simulink model "P1_RC_SIMULINK"  (R2022b)
settings: Solver=VariableStepAuto  StartTime=0.0  StopTime=2.350  RelTol=1e-3
values from neighbouring files (symbols this model uses):
  alpha = (-1)/tau    (= -2.12765957447)    [Main.m]    (also in P1_DINAMICA_SISTEMAS.m)
  beta = 1/tau    (= 2.12765957447)    [Main.m]    (also in P1_DINAMICA_SISTEMAS.m)
  y0 = 2    [Main.m]    (also in P1_DINAMICA_SISTEMAS.m)
settings Model: Creator=zamor  LastModifiedBy=zamor

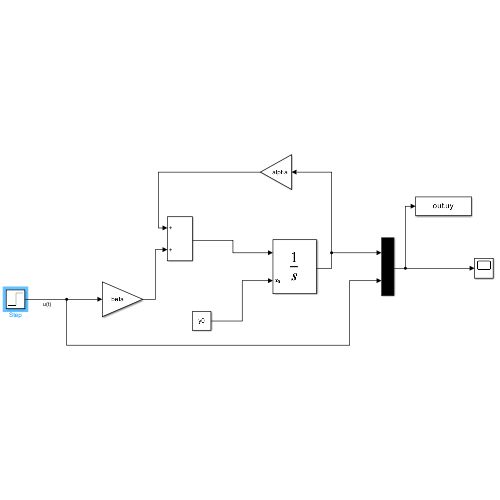
[thumbnail: Simulink's stored preview of the top-level diagram]
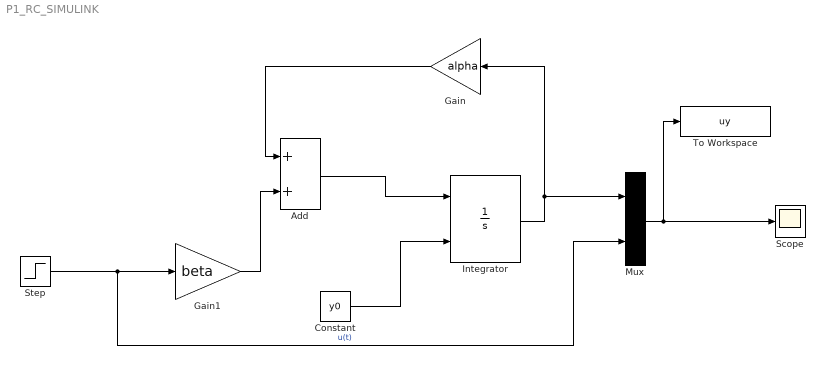
== system P1_RC_SIMULINK ==
  Add : Sum
  Constant : Constant  Value=y0
  Gain : Gain  Gain=alpha
  Gain1 : Gain  Gain=beta
  Integrator : Integrator  InitialConditionSource=external
  Mux : Mux  Inputs=2
  Scope : Scope
  Step : Step  Time=0  SampleTime=0
  To Workspace : ToWorkspace  VariableName=uy  SaveFormat=Timeseries  SampleTime=-1
  wires:
  Add/1 -> Integrator/1
  Constant/1 -> Integrator/2
  Gain1/1 -> Add/2
  Step/1 -> Mux/2, Gain1/1  "u(t)"
  Integrator/1 -> Mux/1, Gain/1
  Gain/1 -> Add/1
  Mux/1 -> Scope/1, To Workspace/1
